simulink model "My_SynchronousMachine_model"  (R2023a)
settings: Solver=ode23t  StartTime=0.0  StopTime=20  RelTol=1e-6
values from neighbouring files (symbols this model uses):
  f = 60    [SynchronousMachineModelParameters.m]
  i_f = Vfd/Rpf    [SynchronousMachineModelParameters.m]
  ids = double(ids)    [SynchronousMachineModelParameters.m]
  iqs = double(iqs)    [SynchronousMachineModelParameters.m]
  J = 35.1e6    (= 35100000)    [SynchronousMachineModelParameters.m]
  JL = Jmat*L    [SynchronousMachineModelParameters.m]
  L = [Lq 0 0 Lmq Lmq 0 0 ... (first row only)    [SynchronousMachineModelParameters.m]
  Linv = inv(L)    [SynchronousMachineModelParameters.m]
  P = 64    [SynchronousMachineModelParameters.m]
  R = [Rs 0 0 0 0 0 0 ... (first row only)    [SynchronousMachineModelParameters.m]
  theta_e0 = theta_r0*P/2    (= 0)    [SynchronousMachineModelParameters.m]
  theta_r0 = 0    [SynchronousMachineModelParameters.m]
  Vabc_s = 20e3*sqrt(2)/sqrt(3)    [SynchronousMachineModelParameters.m]
  Vfd = Epf*Rpf/(Lmd*web)    [SynchronousMachineModelParameters.m]
  wb = 112.5*2*pi/60    (= 11.780972451)    [SynchronousMachineModelParameters.m]
settings Model: Creator=QUDUS  LastModifiedBy=QUDUS

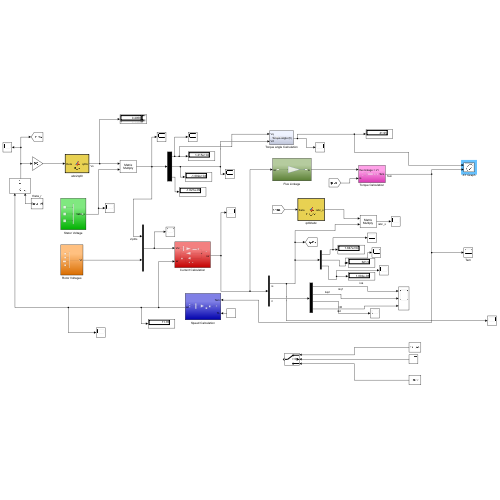
[thumbnail: Simulink's stored preview of the top-level diagram]
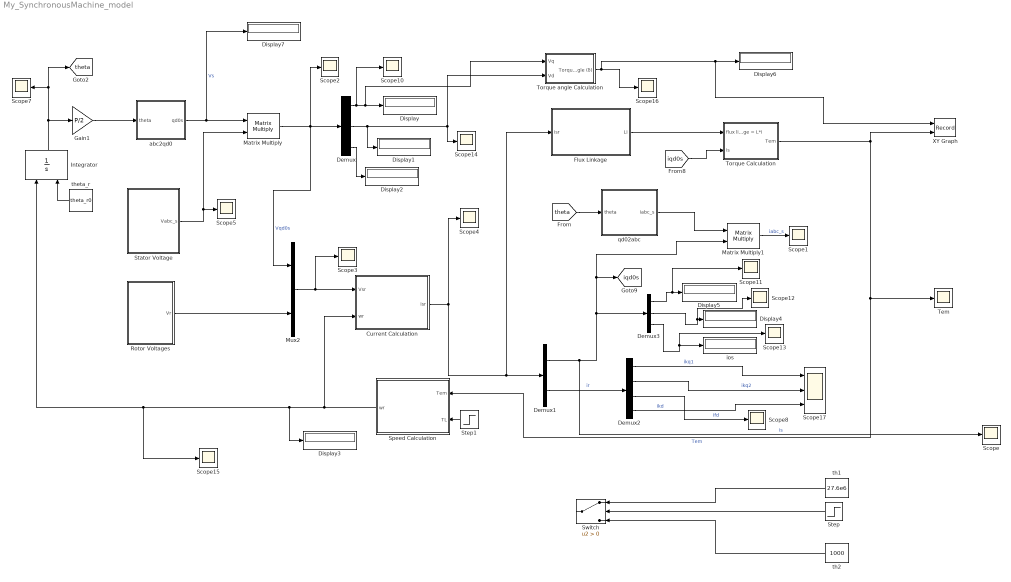
== system My_SynchronousMachine_model ==
  Current Calculation : Subsystem
  Demux : Demux  Outputs=3
  Demux1 : Demux  Outputs=[3 4]
  Demux2 : Demux
  Demux3 : Demux  Outputs=3
  Display{,1..7} (8 alike) : Display
  Flux Linkage : Subsystem
  Gain1 : Gain  Gain=P/2
  Integrator : Integrator  InitialConditionSource=external
  Matrix Multiply : Product  Multiplication=Matrix(*)
  Matrix Multiply1 : Product  Multiplication=Matrix(*)
  Mux2 : Mux  Inputs=[3 4]
  Rotor Voltages : Subsystem
  Scope{,1..5,7..8,10..16} (15 alike) : Scope
  Scope17 : Scope  NumInputPorts=3
  Speed Calculation : Subsystem
  Stator Voltage : Subsystem
  Step : Step  Time=4  SampleTime=0
  Step1 : Step  Time=4  After=27.6e6  SampleTime=0
  Switch : Switch  Criteria=u2 > Threshold  SaturateOnIntegerOverflow=off  InputSameDT=off
  Tem : Scope
  Torque Calculation : Subsystem
  Torque angle Calculation : Subsystem
  XY Graph : Record  FileSettingsInternal="{\"entries\":[{\"content\":{\"excelSettings\":{\"content\":{},\"type\":\"Streamout.ExcelSettings\"}},\"type\":\"Streamout.FileSettingStorage\",\"uuid\":\"\"}],\"packageUris\":[\"http:\\/\\/schema.mathworks.com\\/mf0\\/streamout_blocks\\/R2020a\"],\"version\":\"1.0\"}"  Layout=[1 1]  SignalsInternal="{\"entries\":[{\"content\":{\"signals\":[{\"content\":{\"blockPath\":[],\"dimensions\":[1],\"domain\":\"\",\"lineColor\":\"#a2142f\",\"plots\":[1],\"port\":1,\"sid\":[\"\"],\"signalID\":1996,\"signalName\":\"Torque angle Calculation\"},\"type\":\"RecordBlkView.Signal\",\"uuid\":\"\"},{\"content\":{\"blockPath\":[],\"dimensions\":[1],\"domain\":\"\",\"lineColor\":\"#139fff\",\"plots\":[1],\"port\":2,\"sid\":[\"\"],\"signalID\":2000,\"signalName\":\"Tem\"},\"type\":\"RecordBlkView.Signal\",\"uuid\":\"\"}]},\"type\":\"RecordBlkView.InputSignals\",\"uuid\":\"\"}],\"packageUris\":[\"http:\\/\\/schema.mathworks.com\\/mf0\\/streamout_blocks\\/R2020a\"],\"version\":\"1.0\"}"  VisualizationBindings="{\"xyplotplugin\":{\"info\":[{\"series\":[{\"bindingParametersList\":[{\"parameter\":\"X-Axis\",\"signalID\":1996,\"signalName\":\"Torque angle Calculation\"},{\"parameter\":\"Y-Axis\",\"signalID\":2000,\"signalName\":\"Tem\"}],\"seriesID\":21041}],\"subplotID\":1}]}}"  CompatibilityTag=XY
  abc2qd0 : MATLAB Function  TreatAsAtomicUnit=on
  ios : Display
  qd02abc : MATLAB Function  TreatAsAtomicUnit=on
  th1 : Constant  Value=27.6e6
  th2 : Constant  Value=1000
  theta_r : Constant  Value=theta_r0
  tag scope: iqd0s=global, theta=global
  wires:
  Current Calculation/1(isr) -> Flux Linkage/1(isr), Demux1/1, Scope4/1
  Demux/2 -> Torque angle Calculation/2(Vd), Scope14/1, Display1/1
  Demux/1 -> Scope10/1, Torque angle Calculation/1(Vq), Display/1
  Demux/3 -> Display2/1
  Mux2/1 -> Current Calculation/1(Vsr), Scope3/1
  Matrix Multiply/1 -> Mux2/1, Demux/1, Scope2/1  "Vqd0s"
  qd02abc/1(iabc_s) -> Matrix Multiply1/1
  theta_r/1 -> Integrator/2
  abc2qd0/1(qd0s) -> Display7/1, Matrix Multiply/1  "Vs"
  Rotor Voltages/1(Vr) -> Mux2/2
  Speed Calculation/1(wr) -> Scope15/1, Integrator/1, Display3/1, Current Calculation/2(wr)
  Stator Voltage/1(Vabc_s) -> Matrix Multiply/2, Scope5/1
  Demux3/1 -> Scope11/1, Display5/1
  Demux3/2 -> Scope12/1, Display4/1
  Demux3/3 -> Scope13/1, ios/1
  Demux2/1 -> Scope17/1  "ikq1"
  Demux2/2 -> Scope17/2  "ikq2"
  Demux2/3 -> Scope8/1  "ifd"
  Demux2/4 -> Scope17/3  "ikd"
  [theta] -> qd02abc/1(theta)
  Integrator/1 -> [theta], Scope7/1, Gain1/1
  Demux1/2 -> Demux2/1  "ir"
  Demux1/1 -> Scope/1, Matrix Multiply1/2, [iqd0s], Demux3/1  "is"
  Torque Calculation/1(Tem) -> XY Graph/2, Speed Calculation/1(Tem), Tem/1  "Tem"
  [iqd0s] -> Torque Calculation/2(is)
  Flux Linkage/1(Li) -> Torque Calculation/1(flux linkage = L*i)
  Matrix Multiply1/1 -> Scope1/1  "iabc_s"
  Gain1/1 -> abc2qd0/1(theta)
  Torque angle Calculation/1("Torque angle (δ) ") -> Scope16/1, XY Graph/1, Display6/1
  Step/1 -> Switch/2
  th1/1 -> Switch/1
  th2/1 -> Switch/3
  Step1/1 -> Speed Calculation/2(TL)

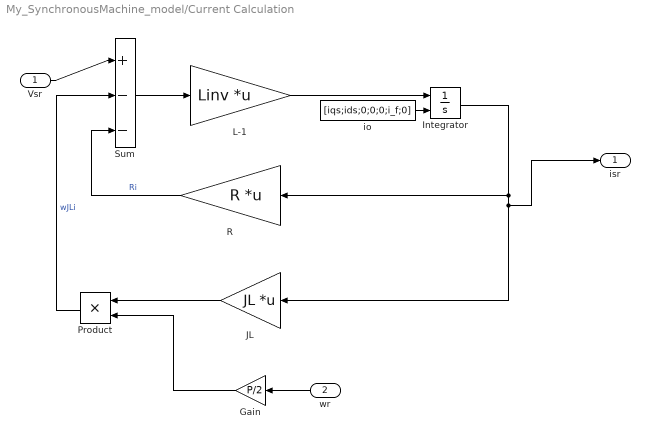
== system My_SynchronousMachine_model/Current Calculation ==
  Vsr : Inport
  wr : Inport  Port=2
  Gain : Gain  Gain=P/2
  Integrator : Integrator  InitialConditionSource=external
  JL : Gain  Gain=JL  Multiplication=Matrix(K*u) (u vector)
  L-1 : Gain  Gain=Linv  Multiplication=Matrix(K*u) (u vector)
  Product : Product
  R : Gain  Gain=R  Multiplication=Matrix(K*u) (u vector)
  Sum : Sum  Inputs=|+--
  io : Constant  Value=[iqs;ids;0;0;0;i_f;0]
  isr : Outport
  wires:
  Vsr/1 -> Sum/1
  Sum/1 -> L-1/1
  R/1 -> Sum/3  "Ri"
  JL/1 -> Product/1
  Product/1 -> Sum/2  "wJLi"
  Integrator/1 -> isr/1, JL/1, R/1
  wr/1 -> Gain/1
  Gain/1 -> Product/2
  L-1/1 -> Integrator/1
  io/1 -> Integrator/2

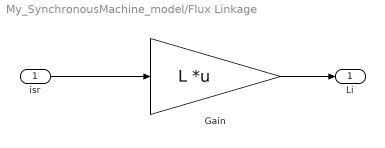
== system My_SynchronousMachine_model/Flux Linkage ==
  isr : Inport
  Gain : Gain  Gain=L  Multiplication=Matrix(K*u) (u vector)
  Li : Outport
  wires:
  Gain/1 -> Li/1
  isr/1 -> Gain/1

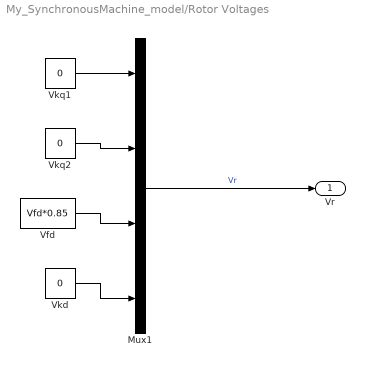
== system My_SynchronousMachine_model/Rotor Voltages ==
  Mux1 : Mux
  Vfd : Constant  Value=Vfd*0.85
  Vkd : Constant  Value=0
  Vkq1 : Constant  Value=0
  Vkq2 : Constant  Value=0
  Vr : Outport
  wires:
  Vkq1/1 -> Mux1/1
  Vkd/1 -> Mux1/4
  Vkq2/1 -> Mux1/2
  Vfd/1 -> Mux1/3
  Mux1/1 -> Vr/1  "Vr"

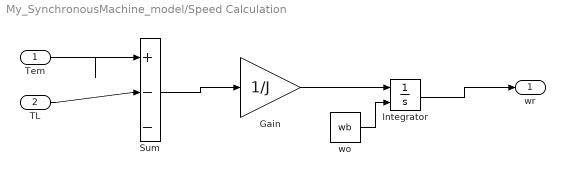
== system My_SynchronousMachine_model/Speed Calculation ==
  Tem : Inport
  TL : Inport  Port=2
  Gain : Gain  Gain=1/J
  Integrator : Integrator  InitialConditionSource=external
  Sum : Sum  Inputs=|+--
  wo : Constant  Value=wb
  wr : Outport
  wires:
  Sum/1 -> Gain/1
  Integrator/1 -> wr/1
  wo/1 -> Integrator/2
  Tem/1 -> Sum/1
  TL/1 -> Sum/2
  Gain/1 -> Integrator/1

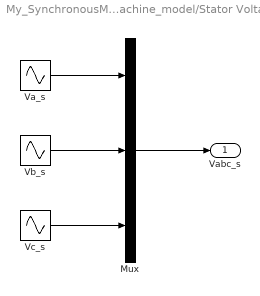
== system My_SynchronousMachine_model/Stator Voltage ==
  Mux : Mux  Inputs=3
  Va_s : Sin  Amplitude=Vabc_s  Frequency=f*2*pi  Phase=theta_e0+pi/2  SampleTime=0
  Vb_s : Sin  Amplitude=Vabc_s  Frequency=f*2*pi  Phase=theta_e0-2*pi/3+pi/2  SampleTime=0
  Vc_s : Sin  Amplitude=Vabc_s  Frequency=f*2*pi  Phase=theta_e0-4*pi/3+pi/2  SampleTime=0
  Vabc_s : Outport
  wires:
  Vc_s/1 -> Mux/3
  Vb_s/1 -> Mux/2
  Va_s/1 -> Mux/1
  Mux/1 -> Vabc_s/1

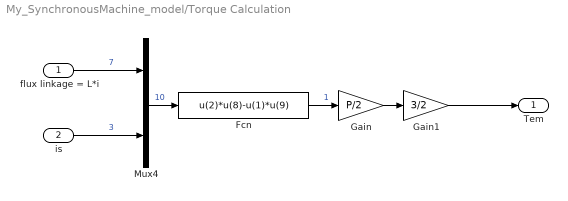
== system My_SynchronousMachine_model/Torque Calculation ==
  flux linkage = L*i : Inport
  is : Inport  Port=2
  Fcn : Fcn  Expr=u(2)*u(8)-u(1)*u(9)
  Gain : Gain  Gain=P/2
  Gain1 : Gain  Gain=3/2
  Mux4 : Mux  Inputs=[7 3]
  Tem : Outport
  wires:
  Gain1/1 -> Tem/1
  Gain/1 -> Gain1/1
  Mux4/1 -> Fcn/1  "10"
  flux linkage = L*i/1 -> Mux4/1  "7"
  Fcn/1 -> Gain/1  "1"
  is/1 -> Mux4/2  "3"

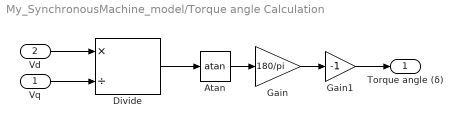
== system My_SynchronousMachine_model/Torque angle Calculation ==
  Vq : Inport
  Vd : Inport  Port=2
  Atan : Trigonometry  Operator=atan
  Divide : Product  Inputs=*/
  Gain : Gain  Gain=180/pi
  Gain1 : Gain  Gain=-1
  "Torque angle (δ) " : Outport
  wires:
  Vd/1 -> Divide/1
  Divide/1 -> Atan/1
  Atan/1 -> Gain/1
  Gain/1 -> Gain1/1
  Vq/1 -> Divide/2
  Gain1/1 -> "Torque angle (δ) "/1

== matlab function My_SynchronousMachine_model/abc2qd0 ==
  data: theta input; qd0s output
function qd0s = K_s(theta)


qd0s= 2/3* [cos(theta) cos(theta-2*pi/3) cos(theta+2*pi/3); sin(theta) sin(theta-2*pi/3) sin(theta+2*pi/3); 1/2 1/2 1/2];

end

== matlab function My_SynchronousMachine_model/qd02abc ==
  data: theta input; iabc_s output
function iabc_s = Ks_inv(theta)


iabc_s= 2/3* [cos(theta) sin(theta) 1; cos(theta-2*pi/3) sin(theta-2*pi/3) 1; cos(theta+2*pi/3) sin(theta+2*pi/3) 1];

end
